simulink model "Diezel_Manual"  (R2019a)
settings: Solver=ode4  StartTime=0.0  StopTime=inf  FixedStep=1e-4  RelTol=1e-2
libraries: simulink_extras x1, simulink x1
settings Model: Creator=anmay  LastModifiedBy=anmay

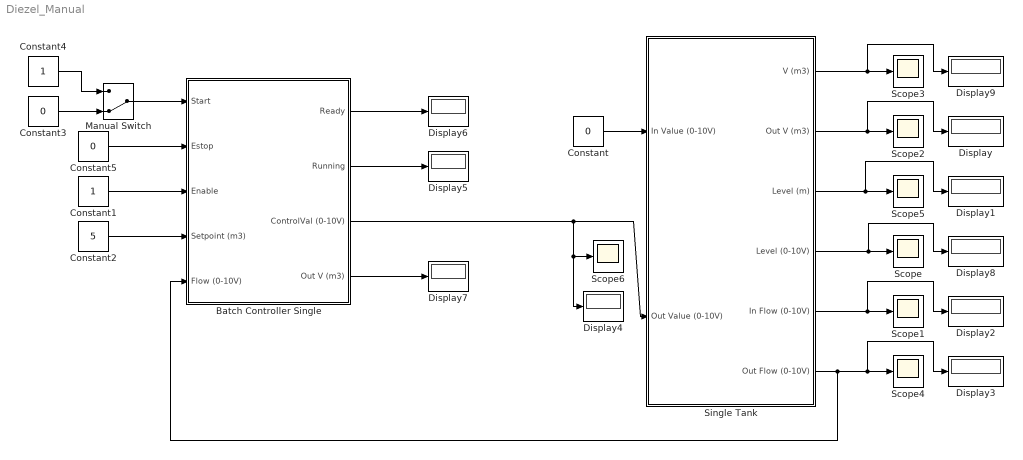
== system Diezel_Manual ==
  Batch Controller Single : Subsystem  mask{FlowMax=200}
      mask prompts: FlowMax "Lưu lượng tối đa (van mở 100%) (l/s)"
  Constant : Constant  Value=0
  Constant1 : Constant
  Constant2 : Constant  Value=5
  Constant3 : Constant  Value=0
  Constant4 : Constant
  Constant5 : Constant  Value=0
  Display{,1..9} (10 alike) : Display
  Manual Switch : ManualSwitch  CurrentSetting=0
  Scope{,1..6} (7 alike) : Scope
  Single Tank : Subsystem  mask{InitialLevel=20, TankHeight=25, FlowMax=200, BaseArea=10, Tqt=0.2, EnableNoise=on, VarNoise=20}
      mask prompts: InitialLevel "Mức nhiên liệu ban đầu (m)"; TankHeight "Chiều cao của bể (m)"; FlowMax "Lưu lượng tối đa (van mở 100%) (l/s)"; BaseArea "Diện tích đáy (m2)"; Tqt "Hằng số quán tính của van (s)"; EnableNoise "Tạo nhiễu"; VarNoise "Phương sai của bộ tạo nhiễu"
  wires:
  Single Tank/1(V (m3)) -> Display9/1, Scope3/1
  Single Tank/2(Out V (m3)) -> Scope2/1, Display/1
  Single Tank/3(Level (m)) -> Scope5/1, Display1/1
  Single Tank/6(Out Flow (0-10V)) -> Batch Controller Single/5(Flow (0-10V)), Display3/1, Scope4/1
  Batch Controller Single/3(ControlVal (0-10V)) -> Display4/1, Scope6/1, Single Tank/2(Out Value (0-10V))
  Batch Controller Single/2(Running) -> Display5/1
  Single Tank/4(Level (0-10V)) -> Scope/1, Display8/1
  Batch Controller Single/1(Ready) -> Display6/1
  Batch Controller Single/4(Out V (m3)) -> Display7/1
  Single Tank/5(In Flow (0-10V)) -> Display2/1, Scope1/1
  Constant/1 -> Single Tank/1(In Value (0-10V))
  Constant1/1 -> Batch Controller Single/3(Enable)
  Constant2/1 -> Batch Controller Single/4(Setpoint (m3))
  Manual Switch/1 -> Batch Controller Single/1(Start)
  Constant3/1 -> Manual Switch/2
  Constant4/1 -> Manual Switch/1
  Constant5/1 -> Batch Controller Single/2(Estop)

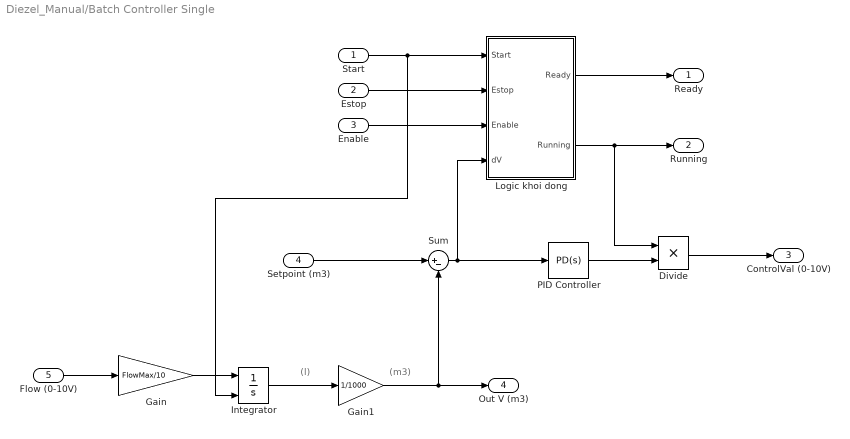
== system Diezel_Manual/Batch Controller Single ==
  note: (m3)
  note: (l)
  Start : Inport
  Estop : Inport  Port=2
  Enable : Inport  Port=3
  Setpoint (m3) : Inport  Port=4
  Flow (0-10V) : Inport  Port=5
  Divide : Product  Inputs=**
  Gain : Gain  Gain=FlowMax/10
  Gain1 : Gain  Gain=1/1000
  Integrator : Integrator  ExternalReset=rising
  Logic khoi dong : Subsystem
  PID Controller : simulink/Continuous/PID Controller  Controller=PD  Form=Parallel  TimeDomain=Continuous-time  SampleTime=-1  IntegratorMethod=Forward Euler  FilterMethod=Forward Euler  ControllerParametersSource=internal  P=30  I=0.5  D=0.5  UseFilter=on  N=100  TunerSelectOption=Transfer Function Based (PID Tuner App)  InitialConditionSource=internal  InitialConditionForIntegrator=0  InitialConditionForFilter=0  DifferentiatorICPrevScaledInput=0  ExternalReset=none  TrackingMode=off  Kt=1  LimitOutput=on  UpperSaturationLimit=10  LowerSaturationLimit=0  LinearizeAsGain=on  AntiWindupMode=clamping  Kb=1  POutMin=[]  POutMax=[]  IOutMin=[]  IOutMax=[]  DOutMin=[]  DOutMax=[]  NOutMin=[]  NOutMax=[]  SumOutMin=[]  SumOutMax=[]  SaturationOutMin=[]  SaturationOutMax=[]  PParamMin=[]  PParamMax=[]  IParamMin=[]  IParamMax=[]  DParamMin=[]  DParamMax=[]  NParamMin=[]  NParamMax=[]  KbParamMin=[]  KbParamMax=[]  KtParamMin=[]  KtParamMax=[]  KbOutMin=[]  KbOutMax=[]  KtOutMin=[]  KtOutMax=[]  IntegratorOutMin=[]  IntegratorOutMax=[]  FilterOutMin=[]  FilterOutMax=[]  SumI1OutMin=[]  SumI1OutMax=[]  SumI2OutMin=[]  SumI2OutMax=[]  SumI3OutMin=[]  SumI3OutMax=[]  SumI4OutMin=[]  SumI4OutMax=[]  SumDOutMin=[]  SumDOutMax=[]  DifferentiatorOutMin=[]  DifferentiatorOutMax=[]  FilterDiffOutCoefMin=[]  FilterDiffOutCoefMax=[]  ReciprocalOutMin=[]  ReciprocalOutMax=[]  SumDenOutMin=[]  SumDenOutMax=[]  SumNumOutMin=[]  SumNumOutMax=[]  DivideOutMin=[]  DivideOutMax=[]  IntegratorContinuousStateAttributes=''  IntegratorStateMustResolveToSignalObject=off  IntegratorRTWStateStorageClass=Auto  FilterContinuousStateAttributes=''  FilterStateMustResolveToSignalObject=off  FilterRTWStateStorageClass=Auto  ParallelPVariant=InternalParameters  IdealPVariant=Disabled  IVariant=Disabled  DVariant=InternalParameters  IntegratorVariant=Disabled  SatVariant=Enabled  AWVariant=Disabled  PCopyVariant=Disabled  TRVariant=Disabled  FdbkBlocksVariant=Forward  IdealPFdbkVariant=Disabled  SatFdbkVariant=Disabled  DerivativeFilterVariant=ContFilter  NVariant=InternalParameters  NCopyVariant=Disabled  FilterICVariant=InternalICsFilter  IntegratorICVariant=Disabled  ExternalResetVariant=Disabled  TRSumVariant=Passthrough  SumFdbkVariant=Disabled  SumVariant=Sum_PD
  Sum : Sum  Inputs=|+-
  Ready : Outport
  Running : Outport  Port=2
  ControlVal (0-10V) : Outport  Port=3
  Out V (m3) : Outport  Port=4
  wires:
  Gain/1 -> Integrator/1
  Flow (0-10V)/1 -> Gain/1
  Sum/1 -> Logic khoi dong/4(dV), PID Controller/1
  Setpoint (m3)/1 -> Sum/1
  Integrator/1 -> Gain1/1
  Divide/1 -> ControlVal (0-10V)/1
  PID Controller/1 -> Divide/2
  Logic khoi dong/2(Running) -> Divide/1, Running/1
  Gain1/1 -> Out V (m3)/1, Sum/2
  Estop/1 -> Logic khoi dong/2(Estop)
  Start/1 -> Integrator/2, Logic khoi dong/1(Start)
  Enable/1 -> Logic khoi dong/3(Enable)
  Logic khoi dong/1(Ready) -> Ready/1

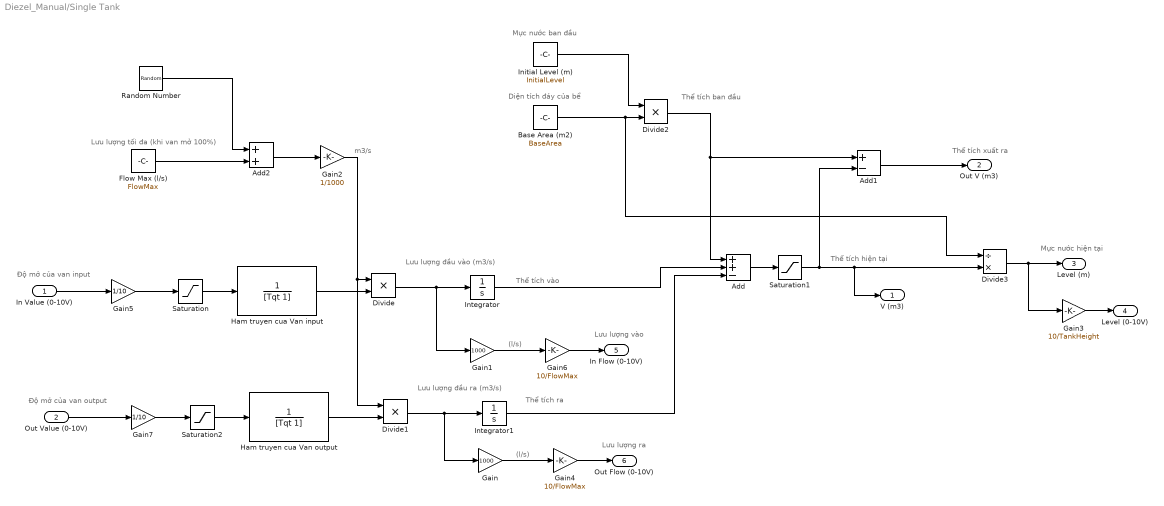
== system Diezel_Manual/Single Tank ==
  note: (l/s)
  note: m3/s
  note: Lưu lượng ra
  note: Thể tích xuất ra
  note: Thể tích hiện tại
  note: Mực nước hiện tại
  note: Thể tích
      | ban đầu
  note: Mực nước ban đầu
  note: Diện tích đáy của bể
  note: Lưu lượng tối đa (khi van mở 100%)
  note: Độ mở của van output
  note: Thể tích ra
  note: Lưu lượng
      | đầu ra (m3/s)
  note: Thể tích vào
  note: Độ mở của van input
  note: Lưu lượng
      | đầu vào (m3/s)
  note: (l/s)
  note: Lưu lượng vào
  In Value (0-10V) : Inport
  Out Value (0-10V) : Inport  Port=2
  Add : Sum  Inputs=++-
  Add1 : Sum  Inputs=+-
  Add2 : Sum
  Base Area (m2) : Constant  Value=BaseArea
  Divide : Product  Inputs=**
  Divide1 : Product  Inputs=**
  Divide2 : Product  Inputs=**
  Divide3 : Product  Inputs=/*
  Flow Max (l/s) : Constant  Value=FlowMax
  Gain : Gain  Gain=1000
  Gain1 : Gain  Gain=1000
  Gain2 : Gain  Gain=1/1000
  Gain3 : Gain  Gain=10/TankHeight
  Gain4 : Gain  Gain=10/FlowMax
  Gain5 : Gain  Gain=1/10
  Gain6 : Gain  Gain=10/FlowMax
  Gain7 : Gain  Gain=1/10
  Ham truyen cua Van input : TransferFcn  Denominator=[Tqt 1]
  Ham truyen cua Van output : TransferFcn  Denominator=[Tqt 1]
  Initial Level (m) : Constant  Value=InitialLevel
  Integrator : Integrator
  Integrator1 : Integrator
  "Random Number " : RandomNumber  Variance=VarNoise*EnableNoise  SampleTime=0.5
  Saturation : Saturate  UpperLimit=1  LowerLimit=0
  Saturation1 : Saturate  UpperLimit=TankHeight*BaseArea  LowerLimit=0
  Saturation2 : Saturate  UpperLimit=1  LowerLimit=0
  V (m3) : Outport
  Out V (m3) : Outport  Port=2
  Level (m) : Outport  Port=3
  Level (0-10V) : Outport  Port=4
  In Flow (0-10V) : Outport  Port=5
  Out Flow (0-10V) : Outport  Port=6
  wires:
  Base Area (m2)/1 -> Divide3/1, Divide2/2
  Initial Level (m)/1 -> Divide2/1
  Divide3/1 -> Gain3/1, Level (m)/1
  Divide2/1 -> Add1/1, Add/1
  Add/1 -> Saturation1/1
  Saturation1/1 -> Add1/2, V (m3)/1, Divide3/2
  Add1/1 -> Out V (m3)/1
  Saturation2/1 -> Ham truyen cua Van output/1
  Ham truyen cua Van output/1 -> Divide1/2
  Divide1/1 -> Gain/1, Integrator1/1
  Gain3/1 -> Level (0-10V)/1
  Gain4/1 -> Out Flow (0-10V)/1
  Gain/1 -> Gain4/1
  Gain7/1 -> Saturation2/1
  Out Value (0-10V)/1 -> Gain7/1
  "Random Number "/1 -> Add2/1
  Add2/1 -> Gain2/1
  Flow Max (l/s)/1 -> Add2/2
  Integrator/1 -> Add/2
  Gain2/1 -> Divide1/1, Divide/1
  Ham truyen cua Van input/1 -> Divide/2
  Saturation/1 -> Ham truyen cua Van input/1
  Gain5/1 -> Saturation/1
  In Value (0-10V)/1 -> Gain5/1
  Integrator1/1 -> Add/3
  Divide/1 -> Gain1/1, Integrator/1
  Gain6/1 -> In Flow (0-10V)/1
  Gain1/1 -> Gain6/1

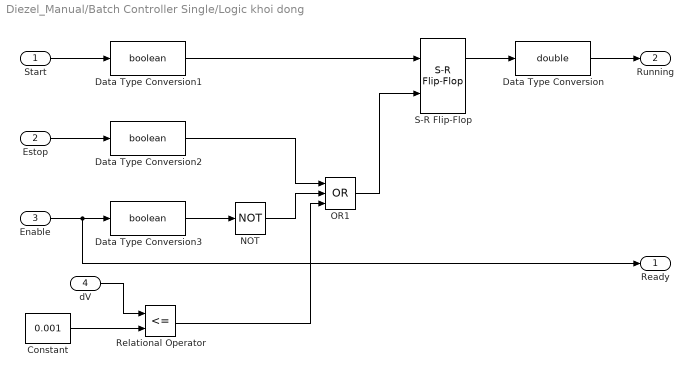
== system Diezel_Manual/Batch Controller Single/Logic khoi dong ==
  Start : Inport
  Estop : Inport  Port=2
  Enable : Inport  Port=3
  dV : Inport  Port=4
  Constant : Constant  Value=0.001
  Data Type Conversion : DataTypeConversion  OutDataTypeStr=double
  Data Type Conversion1 : DataTypeConversion  OutDataTypeStr=boolean
  Data Type Conversion2 : DataTypeConversion  OutDataTypeStr=boolean
  Data Type Conversion3 : DataTypeConversion  OutDataTypeStr=boolean
  NOT : Logic  Operator=NOT  IconShape=distinctive  AllPortsSameDT=off  OutDataTypeStr=boolean
  OR1 : Logic  Operator=OR  Inputs=3  IconShape=distinctive  AllPortsSameDT=off  OutDataTypeStr=boolean
  Relational Operator : RelationalOperator  Operator=<=  OutDataTypeStr=boolean  RndMeth=Simplest
  S-R Flip-Flop : simulink_extras/Flip Flops/S-R Flip-Flop  initial_condition=0
  Ready : Outport
  Running : Outport  Port=2
  wires:
  Constant/1 -> Relational Operator/2
  dV/1 -> Relational Operator/1
  Start/1 -> Data Type Conversion1/1
  Estop/1 -> Data Type Conversion2/1
  Data Type Conversion2/1 -> OR1/1
  Data Type Conversion1/1 -> S-R Flip-Flop/1
  OR1/1 -> S-R Flip-Flop/2
  Data Type Conversion3/1 -> NOT/1
  NOT/1 -> OR1/2
  Relational Operator/1 -> OR1/3
  S-R Flip-Flop/1 -> Data Type Conversion/1
  Data Type Conversion/1 -> Running/1
  Enable/1 -> Ready/1, Data Type Conversion3/1
